simulink model "Model32"  (R2020a)
settings: Solver=VariableStepAuto  StartTime=0.0  StopTime=10.0  RelTol=1e-3
settings Model: Creator=HP  LastModifiedBy=HP

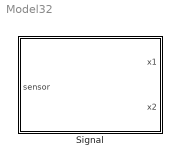
== system Model32 ==
  Signal : Stateflow chart  TreatAsAtomicUnit=on

== stateflow chart Model32/Signal ==
  state Stop
    x1 = RED;
    x2 = GREEN;
  state StopForTraffic
    x1 = RED;
    x2 = GREEN;
  state StopToGo
    x1 = RED;
    x2 = YELLOW;
  state GoToStop
    x1 = YELLOW;
    x2 = RED;
  state Go
    x1 = GREEN;
    x2 = RED;
  (default) -> Stop
  StopForTraffic -> StopToGo : [sensor]
  Stop -> StopForTraffic : after(20,tick)
  GoToStop -> Stop : after (3,tick)
  StopToGo -> Go : after(3,tick)
  Go -> GoToStop : after(10,tick)
  data: x1 output; x2 output; YELLOW constant double; RED constant double; GREEN constant double; sensor input
